simulink model "APP_MyApplication"  (R2018b)
settings: Solver=VariableStepDiscrete  StartTime=0.0  StopTime=10  RelTol=1e-3
PreLoadFcn:
  | if(exist('MBDS_ModelCallback', 'file')), MBDS_ModelCallback('PreLoad'); end;
PostLoadFcn:
  | if(exist('MBDS_ModelCallback', 'file')), MBDS_ModelCallback('PostLoad'); end;
InitFcn:
  | if(exist('MBDS_ModelCallback', 'file')), MBDS_ModelCallback('Init'); end;
StartFcn:
  | if(exist('MBDS_ModelCallback', 'file')), MBDS_ModelCallback('Start'); end;
StopFcn:
  | if(exist('MBDS_ModelCallback', 'file')), MBDS_ModelCallback('Stop'); end;
undefined symbols (not defined in the file): sigbuilder_block, Ts
libraries: KIBES_Signal x499, simulink x8
(part 10 of 10)

== system APP_MyApplication/Model/APP_MyApplication_/DateTime/DateTimeAssemble1/ConvertToNrOfDays/AddDaysForCompleteYears ==
  note: count leap days since 1970
  note: add days for complete years
  u16_Year : Inport  OutDataTypeStr=uint16
  Add : Sum  Inputs=+-  OutDataTypeStr=uint16
  Add1 : Sum  OutDataTypeStr=uint16
  Constant : Constant  Value=1970  OutDataTypeStr=uint16
  Constant1 : Constant  Value=365  OutDataTypeStr=uint16
  Constant2 : Constant  Value=1968  OutDataTypeStr=uint16
  Constant3 : Constant  Value=4  OutDataTypeStr=uint16
  Divide : Product  Inputs=*/  OutDataTypeStr=uint16
  Product : Product  OutDataTypeStr=uint16
  Subtract : Sum  Inputs=+-  OutDataTypeStr=uint16
  u16_DaysForYears : Outport  OutDataTypeStr=uint16
  wires:
  u16_Year/1 -> Subtract/1, Add/1
  Constant/1 -> Add/2
  Add/1 -> Product/1
  Constant1/1 -> Product/2
  Constant2/1 -> Subtract/2
  Subtract/1 -> Divide/1
  Constant3/1 -> Divide/2
  Product/1 -> Add1/1
  Divide/1 -> Add1/2
  Add1/1 -> u16_DaysForYears/1

== system APP_MyApplication/Model/APP_MyApplication_/DateTime/DateTimeAssemble1/ConvertToNrOfDays/CheckIfDateInLeapYearBeforeMarch ==
  note: check if the date is in leap year and before the leap day
  u8_Month : Inport  OutDataTypeStr=uint8
  u16_Year : Inport  Port=2  OutDataTypeStr=uint16
  Constant2 : Constant  Value=1968  OutDataTypeStr=uint16
  Constant3 : Constant  Value=4  OutDataTypeStr=uint16
  Constant6 : Constant  Value=0  OutDataTypeStr=uint16
  Constant7 : Constant  Value=2  OutDataTypeStr=uint8
  Logical Operator : Logic  AllPortsSameDT=off  OutDataTypeStr=boolean
  Math Function : Math  Operator=rem  OutputSignalType=real  SaturateOnIntegerOverflow=on
  Relational Operator1 : RelationalOperator  Operator===  OutDataTypeStr=boolean  RndMeth=Nearest  InputSameDT=on
  Relational Operator3 : RelationalOperator  Operator=<=  OutDataTypeStr=boolean  RndMeth=Nearest
  Subtract : Sum  Inputs=+-  OutDataTypeStr=uint16
  bo_MinusOne : Outport  OutDataTypeStr=boolean
  wires:
  u16_Year/1 -> Subtract/1
  Constant2/1 -> Subtract/2
  Subtract/1 -> Math Function/1
  Constant3/1 -> Math Function/2
  Math Function/1 -> Relational Operator1/1
  Constant6/1 -> Relational Operator1/2
  Constant7/1 -> Relational Operator3/2
  Relational Operator1/1 -> Logical Operator/1
  Relational Operator3/1 -> Logical Operator/2
  u8_Month/1 -> Relational Operator3/1
  Logical Operator/1 -> bo_MinusOne/1

== system APP_MyApplication/Model/APP_MyApplication_/DateTime/DateTimeDisassemble/CheckLeapYearsAndRemainingDays/CalculateLeapYearsSince1970 ==
  u16_NrOfDays : Inport  OutDataTypeStr=uint16
  u16_DaysPerCommonYear : Inport  Port=2  OutDataTypeStr=uint16
  Add : Sum  OutDataTypeStr=uint16
  Constant : Constant  OutDataTypeStr=uint16
  Constant1 : Constant  Value=4  OutDataTypeStr=uint16
  Divide : Product  Inputs=*/  OutDataTypeStr=uint16
  Divide1 : Product  Inputs=*/  OutDataTypeStr=uint16
  u16_NrOfLeapYears : Outport  OutDataTypeStr=uint16
  u16_TempYear : Outport  Port=2  OutDataTypeStr=uint16
  wires:
  Divide/1 -> Add/1, u16_TempYear/1
  Constant/1 -> Add/2
  Constant1/1 -> Divide1/2
  Add/1 -> Divide1/1
  Divide1/1 -> u16_NrOfLeapYears/1
  u16_NrOfDays/1 -> Divide/1
  u16_DaysPerCommonYear/1 -> Divide/2

== system APP_MyApplication/Model/APP_MyApplication_/DateTime/DateTimeDisassemble/CheckLeapYearsAndRemainingDays/CalculateRemainingDays ==
  bo_IsCorrectedYearLeapYear : Inport  OutDataTypeStr=boolean
  bo_IsTempYearCorrect : Inport  Port=2  OutDataTypeStr=boolean
  u16_TempRemainingDays : Inport  Port=3  OutDataTypeStr=uint16
  u16_NrOfLeapYears : Inport  Port=4  OutDataTypeStr=uint16
  u16_DaysPerCommonYear : Inport  Port=5  OutDataTypeStr=uint16
  Add : Sum  OutDataTypeStr=uint16
  Add1 : Sum  Inputs=++-  OutDataTypeStr=uint16
  Constant : Constant  OutDataTypeStr=uint16
  Subtract : Sum  Inputs=+-  OutDataTypeStr=uint16  SaturateOnIntegerOverflow=on
      settings: AttributesFormatString=Saturate: %<SaturateOnIntegerOverflow>
  Switch : Switch  Criteria=u2 ~= 0  OutDataTypeStr=uint16
  Switch1 : Switch  Criteria=u2 ~= 0  OutDataTypeStr=uint16
  u16_TempDate : Outport  OutDataTypeStr=uint16
  wires:
  u16_TempRemainingDays/1 -> Add1/1, Subtract/1
  u16_NrOfLeapYears/1 -> Add1/3, Subtract/2
  u16_DaysPerCommonYear/1 -> Add1/2
  Constant/1 -> Add/1
  bo_IsCorrectedYearLeapYear/1 -> Switch1/2
  Add1/1 -> Add/2, Switch1/3
  Add/1 -> Switch1/1
  Switch1/1 -> Switch/3
  Switch/1 -> u16_TempDate/1
  bo_IsTempYearCorrect/1 -> Switch/2
  Subtract/1 -> Switch/1

== system APP_MyApplication/Model/APP_MyApplication_/DateTime/DateTimeDisassemble/CheckLeapYearsAndRemainingDays/CheckIfCorrectedTempYearIsLeap ==
  u16_CorrectedTempYear : Inport  OutDataTypeStr=uint16
  Add : Sum  OutDataTypeStr=uint16
  Constant : Constant  Value=2  OutDataTypeStr=uint16
  Constant1 : Constant  Value=4  OutDataTypeStr=uint16
  Constant2 : Constant  Value=0  OutDataTypeStr=uint16
  Math Function : Math  Operator=rem  OutputSignalType=real  SaturateOnIntegerOverflow=on
  Relational Operator : RelationalOperator  Operator===  OutDataTypeStr=boolean  RndMeth=Nearest
  bo_IsCorrectedYearLeapYear : Outport  OutDataTypeStr=boolean
  wires:
  u16_CorrectedTempYear/1 -> Add/1
  Add/1 -> Math Function/1
  Math Function/1 -> Relational Operator/1
  Constant/1 -> Add/2
  Constant1/1 -> Math Function/2
  Constant2/1 -> Relational Operator/2
  Relational Operator/1 -> bo_IsCorrectedYearLeapYear/1

== system APP_MyApplication/Model/APP_MyApplication_/DateTime/DateTimeDisassemble/CheckLeapYearsAndRemainingDays/CheckIfTempYearIsCorrect ==
  u16_TempRemainingDays : Inport  OutDataTypeStr=uint16
  u16_NrOfLeapYears : Inport  Port=2  OutDataTypeStr=uint16
  Relational Operator : RelationalOperator  OutDataTypeStr=boolean  RndMeth=Nearest
  bo_IsTempYearCorrect : Outport  OutDataTypeStr=boolean
  wires:
  u16_TempRemainingDays/1 -> Relational Operator/1
  u16_NrOfLeapYears/1 -> Relational Operator/2
  Relational Operator/1 -> bo_IsTempYearCorrect/1

== system APP_MyApplication/Model/APP_MyApplication_/DateTime/DateTimeDisassemble/CheckLeapYearsAndRemainingDays/CheckLeapYear ==
  note: check if the current year is a leap year
  u16_Year : Inport  OutDataTypeStr=uint16
  Add6 : Sum  OutDataTypeStr=uint16
  Constant : Constant  Value=2  OutDataTypeStr=uint8
  Constant1 : Constant  Value=4  OutDataTypeStr=uint16
  Constant9 : Constant  Value=0  OutDataTypeStr=uint16
  Math Function : Math  Operator=rem  OutputSignalType=real  SaturateOnIntegerOverflow=on
  Relational Operator2 : RelationalOperator  Operator===  OutDataTypeStr=boolean  RndMeth=Nearest  InputSameDT=on
  bo_LeapYear : Outport  OutDataTypeStr=boolean
  wires:
  Add6/1 -> Math Function/1
  Relational Operator2/1 -> bo_LeapYear/1
  u16_Year/1 -> Add6/1
  Math Function/1 -> Relational Operator2/1
  Constant9/1 -> Relational Operator2/2
  Constant/1 -> Add6/2
  Constant1/1 -> Math Function/2

== system APP_MyApplication/Model/APP_MyApplication_/DateTime/DateTimeDisassemble/ConvertToMonthAndDay/CheckNrOfDaysInNextMonth ==
  u8_DaysPerMonth : Inport  OutDataTypeStr=uint8
  i8_IterationNr : Inport  Port=2  OutDataTypeStr=int8
  bo_LeapYear : Inport  Port=3  OutDataTypeStr=boolean
  Add1 : Sum  OutDataTypeStr=uint8
  CheckNextMonthFebLeapYear : Subsystem
  Selector : Selector  IndexMode=Zero-based  InputPortWidth=13  IndexOptions=Index vector (port)  Indices=[1 3]  OutputSizes=1
  u8_DaysInNextMonth : Outport  OutDataTypeStr=uint8
  wires:
  bo_LeapYear/1 -> CheckNextMonthFebLeapYear/2(bo_LeapYear)
  i8_IterationNr/1 -> Selector/2, CheckNextMonthFebLeapYear/1(i8_IterationNr)
  u8_DaysPerMonth/1 -> Selector/1
  Selector/1 -> Add1/1
  CheckNextMonthFebLeapYear/1(bo_IsNextFebLeapYear) -> Add1/2
  Add1/1 -> u8_DaysInNextMonth/1

== system APP_MyApplication/Model/APP_MyApplication_/DateTime/DateTimeDisassemble/ConvertToMonthAndDay/SubstractDaysOfMonths ==
  u16_TempDate : Inport  OutDataTypeStr=uint16
  bo_LeapYear : Inport  Port=2  OutDataTypeStr=boolean
  i8_IterationNr : Inport  Port=3  OutDataTypeStr=int8
  u8_DaysPerMonth : Inport  Port=4  OutDataTypeStr=uint8
  Add : Sum  OutDataTypeStr=uint16
  Add1 : Sum  OutDataTypeStr=uint16
  Add2 : Sum  Inputs=+-  OutDataTypeStr=uint8
  CheckCurrMonthFebLeapYear : Subsystem
  Constant : Constant  OutDataTypeStr=int8
  Selector : Selector  IndexMode=Zero-based  InputPortWidth=13  IndexOptions=Index vector (port)  Indices=[1 3]  OutputSizes=1
  Subtract : Sum  Inputs=+-  OutDataTypeStr=uint16
  Unit Delay : UnitDelay  SampleTime=-1
  u16_RemainingDays : Outport  OutDataTypeStr=uint16
  wires:
  bo_LeapYear/1 -> CheckCurrMonthFebLeapYear/1(bo_LeapYear)
  i8_IterationNr/1 -> Add2/1, CheckCurrMonthFebLeapYear/2(i8_IterationNr)
  u8_DaysPerMonth/1 -> Selector/1
  u16_TempDate/1 -> Subtract/1
  Subtract/1 -> u16_RemainingDays/1
  CheckCurrMonthFebLeapYear/1(bo_IsCurrFebLeapYear) -> Add/1
  Selector/1 -> Add/2
  Add/1 -> Add1/1
  Add1/1 -> Subtract/2, Unit Delay/1
  Unit Delay/1 -> Add1/2
  Add2/1 -> Selector/2
  Constant/1 -> Add2/2

== system APP_MyApplication/Model/APP_MyApplication_/DateTime/DateTimeDisassemble/ConvertToTimeAndNrOfDays/CalculateHours ==
  note: 24 hrs/d
  u32_TempDateHrs : Inport  OutDataTypeStr=uint32
  Constant : Constant  Value=24  OutDataTypeStr=uint32
  Data Type Conversion : DataTypeConversion  OutDataTypeStr=uint8
  Data Type Conversion1 : DataTypeConversion  OutDataTypeStr=uint16
  Divide : Product  Inputs=*/  OutDataTypeStr=uint32
  Math Function : Math  Operator=rem  OutputSignalType=real  SaturateOnIntegerOverflow=on
  u8_Hours : Outport  OutDataTypeStr=uint8
  u16_NrOfDays : Outport  Port=2  OutDataTypeStr=uint16
  wires:
  Math Function/1 -> Data Type Conversion/1
  Data Type Conversion/1 -> u8_Hours/1
  Divide/1 -> Data Type Conversion1/1
  Data Type Conversion1/1 -> u16_NrOfDays/1
  Constant/1 -> Math Function/2, Divide/2
  u32_TempDateHrs/1 -> Divide/1, Math Function/1

== system APP_MyApplication/Model/APP_MyApplication_/DateTime/DateTimeDisassemble/ConvertToTimeAndNrOfDays/CalculateMinutes ==
  note: 60 min/h
  u32_TempDateMin : Inport  OutDataTypeStr=uint32
  Constant1 : Constant  Value=60  OutDataTypeStr=uint32
  Data Type Conversion1 : DataTypeConversion  OutDataTypeStr=uint8
  Divide : Product  Inputs=*/  OutDataTypeStr=uint32
  Math Function : Math  Operator=rem  OutputSignalType=real  SaturateOnIntegerOverflow=on
  u8_Minutes : Outport  OutDataTypeStr=uint8
  u32_TempDateHrs : Outport  Port=2  OutDataTypeStr=uint32
  wires:
  Math Function/1 -> Data Type Conversion1/1
  u32_TempDateMin/1 -> Divide/1, Math Function/1
  Divide/1 -> u32_TempDateHrs/1
  Constant1/1 -> Math Function/2, Divide/2
  Data Type Conversion1/1 -> u8_Minutes/1

== system APP_MyApplication/Model/APP_MyApplication_/DateTime/DateTimeDisassemble/ConvertToTimeAndNrOfDays/CalculateSeconds ==
  note: 60 sec/min
  u32_TimeInSeconds : Inport  OutDataTypeStr=uint32
  Constant : Constant  Value=60  OutDataTypeStr=uint32
  Data Type Conversion : DataTypeConversion  OutDataTypeStr=uint8
  Divide : Product  Inputs=*/  OutDataTypeStr=uint32
  Math Function : Math  Operator=rem  OutputSignalType=real  SaturateOnIntegerOverflow=on
  u8_Seconds : Outport  OutDataTypeStr=uint8
  u32_TempDateMin : Outport  Port=2  OutDataTypeStr=uint32
  wires:
  u32_TimeInSeconds/1 -> Divide/1, Math Function/1
  Math Function/1 -> Data Type Conversion/1
  Data Type Conversion/1 -> u8_Seconds/1
  Constant/1 -> Divide/2, Math Function/2
  Divide/1 -> u32_TempDateMin/1

== system APP_MyApplication/Model/APP_MyApplication_/EEProm/TimerPulse/EdgeRising/NoReset ==
  Unused1 : Inport
  Unused2 : Inport  Port=2
  u : Inport  Port=3
  Terminator : Terminator
  Terminator1 : Terminator
  y : Outport
  wires:
  u/1 -> y/1
  Unused1/1 -> Terminator1/1
  Unused2/1 -> Terminator/1

== system APP_MyApplication/Model/APP_MyApplication_/EEProm/TimerPulse/Timer_RE1/DoubleReset ==
  IV : Inport
  R1 : Inport  Port=2
  R2 : Inport  Port=3
  u : Inport  Port=4
  Logical Operator : Logic  AllPortsSameDT=off  OutDataTypeStr=boolean
  Switch1 : Switch  Criteria=u2 ~= 0  OutDataTypeStr=Inherit: Inherit via back propagation  InputSameDT=on
  y : Outport
  wires:
  u/1 -> Switch1/3
  Switch1/1 -> y/1
  IV/1 -> Switch1/1
  Logical Operator/1 -> Switch1/2
  R1/1 -> Logical Operator/1
  R2/1 -> Logical Operator/2

== system APP_MyApplication/Model/APP_MyApplication_/EEProm/TimerPulse/Timer_RE1/NoEnable ==
  u : Inport
  Unused1 : Inport  Port=2
  Unused2 : Inport  Port=3
  Terminator : Terminator
  Terminator1 : Terminator
  y : Outport
  wires:
  Unused2/1 -> Terminator1/1
  u/1 -> y/1
  Unused1/1 -> Terminator/1

== system APP_MyApplication/Model/APP_MyApplication_/EEProm/TimerPulse1/EdgeRising/NoReset ==
  Unused1 : Inport
  Unused2 : Inport  Port=2
  u : Inport  Port=3
  Terminator : Terminator
  Terminator1 : Terminator
  y : Outport
  wires:
  u/1 -> y/1
  Unused1/1 -> Terminator1/1
  Unused2/1 -> Terminator/1

== system APP_MyApplication/Model/APP_MyApplication_/EEProm/TimerPulse1/Timer_RE1/DoubleReset ==
  IV : Inport
  R1 : Inport  Port=2
  R2 : Inport  Port=3
  u : Inport  Port=4
  Logical Operator : Logic  AllPortsSameDT=off  OutDataTypeStr=boolean
  Switch1 : Switch  Criteria=u2 ~= 0  OutDataTypeStr=Inherit: Inherit via back propagation  InputSameDT=on
  y : Outport
  wires:
  u/1 -> Switch1/3
  Switch1/1 -> y/1
  IV/1 -> Switch1/1
  Logical Operator/1 -> Switch1/2
  R1/1 -> Logical Operator/1
  R2/1 -> Logical Operator/2

== system APP_MyApplication/Model/APP_MyApplication_/EEProm/TimerPulse1/Timer_RE1/NoEnable ==
  u : Inport
  Unused1 : Inport  Port=2
  Unused2 : Inport  Port=3
  Terminator : Terminator
  Terminator1 : Terminator
  y : Outport
  wires:
  Unused2/1 -> Terminator1/1
  u/1 -> y/1
  Unused1/1 -> Terminator/1

== system APP_MyApplication/Model/APP_MyApplication_/DTC/DateTimeDisassemble/ConvertToMonthAndDay/CheckNrOfDaysInNextMonth/CheckNextMonthFebLeapYear ==
  note: check if next month is a February of a leap year
  i8_IterationNr : Inport  OutDataTypeStr=int8
  bo_LeapYear : Inport  Port=2  OutDataTypeStr=boolean
  Constant : Constant  Value=2  OutDataTypeStr=int8
  Logical Operator : Logic  AllPortsSameDT=off  OutDataTypeStr=boolean
  Relational Operator : RelationalOperator  Operator===  OutDataTypeStr=boolean  RndMeth=Nearest  InputSameDT=on
  bo_IsNextFebLeapYear : Outport  OutDataTypeStr=boolean
  wires:
  Logical Operator/1 -> bo_IsNextFebLeapYear/1
  Relational Operator/1 -> Logical Operator/1
  bo_LeapYear/1 -> Logical Operator/2
  Constant/1 -> Relational Operator/2
  i8_IterationNr/1 -> Relational Operator/1

== system APP_MyApplication/Model/APP_MyApplication_/DTC/DateTimeDisassemble/ConvertToMonthAndDay/SubstractDaysOfMonths/CheckCurrMonthFebLeapYear ==
  note: check if current month is a February of a leap year
  bo_LeapYear : Inport  OutDataTypeStr=boolean
  i8_IterationNr : Inport  Port=2  OutDataTypeStr=int8
  Constant : Constant  Value=3  OutDataTypeStr=int8
  Logical Operator : Logic  AllPortsSameDT=off  OutDataTypeStr=boolean
  Relational Operator : RelationalOperator  Operator===  OutDataTypeStr=boolean  RndMeth=Nearest  InputSameDT=on
  bo_IsCurrFebLeapYear : Outport  OutDataTypeStr=boolean
  wires:
  Logical Operator/1 -> bo_IsCurrFebLeapYear/1
  Relational Operator/1 -> Logical Operator/2
  bo_LeapYear/1 -> Logical Operator/1
  Constant/1 -> Relational Operator/2
  i8_IterationNr/1 -> Relational Operator/1

== system APP_MyApplication/Model/APP_MyApplication_/DateTime/DateTimeAssemble/CheckIfInputIsValid/CheckIfDayIsValid/CheckIfFebruaryOfLeapYear ==
  note: check if the day is in February of a leap year
  u8_DayIn : Inport  OutDataTypeStr=uint8
  u8_MonthIn : Inport  Port=2  OutDataTypeStr=uint8
  u16_YearIn : Inport  Port=3  OutDataTypeStr=uint16
  Constant : Constant  Value=4  OutDataTypeStr=uint16
  Constant1 : Constant  Value=2  OutDataTypeStr=uint8
  Constant4 : Constant  Value=1968  OutDataTypeStr=uint16
  Constant7 : Constant  Value=29  OutDataTypeStr=uint8
  Data Type Conversion1 : DataTypeConversion  OutDataTypeStr=boolean
  Logical Operator : Logic  Inputs=3  AllPortsSameDT=off  OutDataTypeStr=boolean
  Logical Operator1 : Logic  Operator=NOT  AllPortsSameDT=off  OutDataTypeStr=boolean
  Math Function : Math  Operator=rem  OutputSignalType=real  SaturateOnIntegerOverflow=on
  Relational Operator : RelationalOperator  Operator===  OutDataTypeStr=boolean  RndMeth=Nearest
  Relational Operator1 : RelationalOperator  Operator===  OutDataTypeStr=boolean  RndMeth=Nearest
  Subtract : Sum  Inputs=+-  OutDataTypeStr=uint16  SaturateOnIntegerOverflow=on
      settings: AttributesFormatString=Saturate: %<SaturateOnIntegerOverflow>
  bo_IsFebrauryOfLeapYear : Outport  OutDataTypeStr=boolean
  wires:
  u16_YearIn/1 -> Subtract/1
  u8_MonthIn/1 -> Relational Operator/1
  Constant4/1 -> Subtract/2
  Subtract/1 -> Math Function/1
  Constant7/1 -> Relational Operator1/2
  Relational Operator1/1 -> Logical Operator/1
  Math Function/1 -> Data Type Conversion1/1
  Logical Operator1/1 -> Logical Operator/3
  Constant/1 -> Math Function/2
  u8_DayIn/1 -> Relational Operator1/1
  Constant1/1 -> Relational Operator/2
  Relational Operator/1 -> Logical Operator/2
  Logical Operator/1 -> bo_IsFebrauryOfLeapYear/1
  Data Type Conversion1/1 -> Logical Operator1/1

== system APP_MyApplication/Model/APP_MyApplication_/DateTime/DateTimeAssemble1/CheckIfInputIsValid/CheckIfDayIsValid/CheckIfFebruaryOfLeapYear ==
  note: check if the day is in February of a leap year
  u8_DayIn : Inport  OutDataTypeStr=uint8
  u8_MonthIn : Inport  Port=2  OutDataTypeStr=uint8
  u16_YearIn : Inport  Port=3  OutDataTypeStr=uint16
  Constant : Constant  Value=4  OutDataTypeStr=uint16
  Constant1 : Constant  Value=2  OutDataTypeStr=uint8
  Constant4 : Constant  Value=1968  OutDataTypeStr=uint16
  Constant7 : Constant  Value=29  OutDataTypeStr=uint8
  Data Type Conversion1 : DataTypeConversion  OutDataTypeStr=boolean
  Logical Operator : Logic  Inputs=3  AllPortsSameDT=off  OutDataTypeStr=boolean
  Logical Operator1 : Logic  Operator=NOT  AllPortsSameDT=off  OutDataTypeStr=boolean
  Math Function : Math  Operator=rem  OutputSignalType=real  SaturateOnIntegerOverflow=on
  Relational Operator : RelationalOperator  Operator===  OutDataTypeStr=boolean  RndMeth=Nearest
  Relational Operator1 : RelationalOperator  Operator===  OutDataTypeStr=boolean  RndMeth=Nearest
  Subtract : Sum  Inputs=+-  OutDataTypeStr=uint16  SaturateOnIntegerOverflow=on
      settings: AttributesFormatString=Saturate: %<SaturateOnIntegerOverflow>
  bo_IsFebrauryOfLeapYear : Outport  OutDataTypeStr=boolean
  wires:
  u16_YearIn/1 -> Subtract/1
  u8_MonthIn/1 -> Relational Operator/1
  Constant4/1 -> Subtract/2
  Subtract/1 -> Math Function/1
  Constant7/1 -> Relational Operator1/2
  Relational Operator1/1 -> Logical Operator/1
  Math Function/1 -> Data Type Conversion1/1
  Logical Operator1/1 -> Logical Operator/3
  Constant/1 -> Math Function/2
  u8_DayIn/1 -> Relational Operator1/1
  Constant1/1 -> Relational Operator/2
  Relational Operator/1 -> Logical Operator/2
  Logical Operator/1 -> bo_IsFebrauryOfLeapYear/1
  Data Type Conversion1/1 -> Logical Operator1/1

== system APP_MyApplication/Model/APP_MyApplication_/DateTime/DateTimeDisassemble/ConvertToMonthAndDay/CheckNrOfDaysInNextMonth/CheckNextMonthFebLeapYear ==
  note: check if next month is a February of a leap year
  i8_IterationNr : Inport  OutDataTypeStr=int8
  bo_LeapYear : Inport  Port=2  OutDataTypeStr=boolean
  Constant : Constant  Value=2  OutDataTypeStr=int8
  Logical Operator : Logic  AllPortsSameDT=off  OutDataTypeStr=boolean
  Relational Operator : RelationalOperator  Operator===  OutDataTypeStr=boolean  RndMeth=Nearest  InputSameDT=on
  bo_IsNextFebLeapYear : Outport  OutDataTypeStr=boolean
  wires:
  Logical Operator/1 -> bo_IsNextFebLeapYear/1
  Relational Operator/1 -> Logical Operator/1
  bo_LeapYear/1 -> Logical Operator/2
  Constant/1 -> Relational Operator/2
  i8_IterationNr/1 -> Relational Operator/1

== system APP_MyApplication/Model/APP_MyApplication_/DateTime/DateTimeDisassemble/ConvertToMonthAndDay/SubstractDaysOfMonths/CheckCurrMonthFebLeapYear ==
  note: check if current month is a February of a leap year
  bo_LeapYear : Inport  OutDataTypeStr=boolean
  i8_IterationNr : Inport  Port=2  OutDataTypeStr=int8
  Constant : Constant  Value=3  OutDataTypeStr=int8
  Logical Operator : Logic  AllPortsSameDT=off  OutDataTypeStr=boolean
  Relational Operator : RelationalOperator  Operator===  OutDataTypeStr=boolean  RndMeth=Nearest  InputSameDT=on
  bo_IsCurrFebLeapYear : Outport  OutDataTypeStr=boolean
  wires:
  Logical Operator/1 -> bo_IsCurrFebLeapYear/1
  Relational Operator/1 -> Logical Operator/2
  bo_LeapYear/1 -> Logical Operator/1
  Constant/1 -> Relational Operator/2
  i8_IterationNr/1 -> Relational Operator/1

== stateflow chart APP_MyApplication/Model/APP_MyApplication_/UDS Service/Chart ==
  state Wait
    en:
    u8Response = 120;
  state SendData
    (default) -> (junction 8)
    (junction 8) -> (junction 10) [order 1] : [u8Return==0]
    (junction 8) -> (junction 12) [order 2] : {u8Response = u8Return;}
    (junction 10) -> (junction 15) : {u8Response = 0;}
    (junction 15) -> (junction 12)
    (junction 12) -> (junction 14)
  (default) -> Wait
  SendData -> Wait
  Wait -> SendData : [hasChangedTo(boRequest,1)]
  data: boRequest input boolean; u8Return input uint8; u8Response output uint8
